simulink model "Refined_Model_230322"  (R2020b)
settings: Solver=FixedStepAuto  StartTime=0.0  StopTime=90  FixedStep=dt  RelTol=1e-3
values from neighbouring files (symbols this model uses):
  CovDist = RoadProfile(:,4)    [ICE_Val.m]
  Cx = VehicleDefine(7,3)    [BEV_Basictest.m]    (also in GPS_val.m; ICEBEV_Script.m; ICEBEV_Script_VECTO.m; ICE_Script.m)
  Dist = 1:length(MaxSpeedProfile)    [GPS_val.m]    (also in ICE_Script.m; ICE_Val.m = [1:CovDist(end)])
  dt = 0.1    [GPS_val.m]    (also in ICEBEV_Script.m; ICEBEV_Script_VECTO.m; ICE_Script.m; ICE_Script_SSVal.m)
  DynRolRad = VehicleDefine(5,3)    [BEV_Basictest.m]    (also in GPS_val.m; ICEBEV_Script.m; ICEBEV_Script_VECTO.m; ICE_Script.m)
  EngineRpm = round(IntpTorCur(:,1))    [GPS_val.m]    (also in ICEBEV_Script.m; ICEBEV_Script_VECTO.m; ICE_Script.m; ICE_Script_SSVal.m)
  EngineRpmUse = [EngineRpmUse1; EngineRpmUse2]    [GPS_val.m]    (also in ICEBEV_Script.m; ICEBEV_Script_VECTO.m; ICE_Script.m; ICE_Script_SSVal.m)
  etaClutch = VehicleDefine(23,3)    [GPS_val.m]    (also in ICEBEV_Script.m; ICEBEV_Script_VECTO.m; ICE_Script.m; ICE_Script_SSVal.m)
  etaGRa = GBXDefine(:,3)    [GPS_val.m]    (also in ICEBEV_Script.m; ICEBEV_Script_VECTO.m; ICE_Script.m; ICE_Script_SSVal.m)
  FDR = VehicleDefine(20,3)    [BEV_Basictest.m]    (also in GPS_val.m = VehicleDefine(22,3); ICEBEV_Script.m = VehicleDefine(22,3); ICEBEV_Script_VECTO.m = VehicleDefine(22,3); ICE_Script.m = VehicleDefine(22,3))
  FLoadTor = IntpTorCur(:,2)    [GPS_val.m]    (also in ICEBEV_Script.m; ICEBEV_Script_VECTO.m; ICE_Script.m; ICE_Script_SSVal.m)
  Fr = VehicleDefine(13,3)    [BEV_Basictest.m]    (also in GPS_val.m; ICEBEV_Script.m; ICEBEV_Script_VECTO.m; ICE_Script.m)
  g = VehicleDefine(14,3)    [BEV_Basictest.m]    (also in GPS_val.m; ICEBEV_Script.m; ICEBEV_Script_VECTO.m; ICE_Script.m)
  GNo = GBXDefine(:,1)    [GPS_val.m]    (also in ICEBEV_Script.m; ICEBEV_Script_VECTO.m; ICE_Script.m; ICE_Script_SSVal.m)
  GRa = GBXDefine(:,2)    [GPS_val.m]    (also in ICEBEV_Script.m; ICEBEV_Script_VECTO.m; ICE_Script.m; ICE_Script_SSVal.m)
  IntpSlope = round(IntpSlope,1)    [GPS_val.m]    (also in ICE_Script.m; ICE_Val.m = A)
  Jk = VehicleDefine(15,3)    [BEV_Basictest.m]    (also in GPS_val.m; ICEBEV_Script.m; ICEBEV_Script_VECTO.m; ICE_Script.m)
  Jm = VehicleDefine(16,3)    [GPS_val.m]    (also in ICEBEV_Script.m; ICEBEV_Script_VECTO.m; ICE_Script.m; ICE_Script_SSVal.m)
  MaxSpeedProfile = FMSP    [GPS_val.m]    (also in ICE_Script.m; ICE_Val.m = repelem(SegSPLatinmps,SegLeninm))
  Me = VehicleDefine(10,3)    [BEV_Basictest.m]    (also in GPS_val.m; ICEBEV_Script.m; ICEBEV_Script_VECTO.m; ICE_Script.m)
  MotoringTor = IntpTorCur(:,3)    [GPS_val.m]    (also in ICEBEV_Script.m; ICEBEV_Script_VECTO.m; ICE_Script.m; ICE_Script_SSVal.m)
  Mt = VehicleDefine(12,3)    [BEV_Basictest.m]    (also in GPS_val.m; ICEBEV_Script.m; ICEBEV_Script_VECTO.m; ICE_Script.m)
  Mtot = Mv+Me+Mt    [BEV_Basictest.m]    (also in GPS_val.m; ICEBEV_Script.m; ICEBEV_Script_VECTO.m; ICE_Script.m)
  Mv = VehicleDefine(9,3)    [BEV_Basictest.m]    (also in GPS_val.m; ICEBEV_Script.m; ICEBEV_Script_VECTO.m; ICE_Script.m)
  NoWhlFA = VehicleDefine(2,3)    [BEV_Basictest.m]    (also in GPS_val.m; ICE_Script.m; ICE_Val.m; ICE_Val_new.m)
  NoWhlRA = VehicleDefine(4,3)    [BEV_Basictest.m]    (also in GPS_val.m; ICE_Script.m; ICE_Val.m; ICE_Val_new.m)
  rho = VehicleDefine(6,3)    [BEV_Basictest.m]    (also in GPS_val.m; ICEBEV_Script.m; ICEBEV_Script_VECTO.m; ICE_Script.m)
  SegNo = RoadProfile(:,1)    [ICE_Val.m]
  SegSPLatinmps = (sqrt(aMaxLat*g*CurRadinm))    [GPS_val.m]    (also in ICE_Script.m; ICE_Val.m)
  Sx = VehicleDefine(8,3)    [BEV_Basictest.m]    (also in GPS_val.m; ICEBEV_Script.m; ICEBEV_Script_VECTO.m; ICE_Script.m)
undefined symbols (not defined in the file or in its folder): AccLim, FLoadTorUse, G1Inprpm, GearNo, GInprpm, GInpTor, GTorLoss, MaxSpinG, MaxWhlTorinG
libraries: pid_lib x1
settings Model: Creator=Kshitij  LastModifiedBy=Kshitij
settings SolverCC: AlgebraicLoopSolver=LineSearch

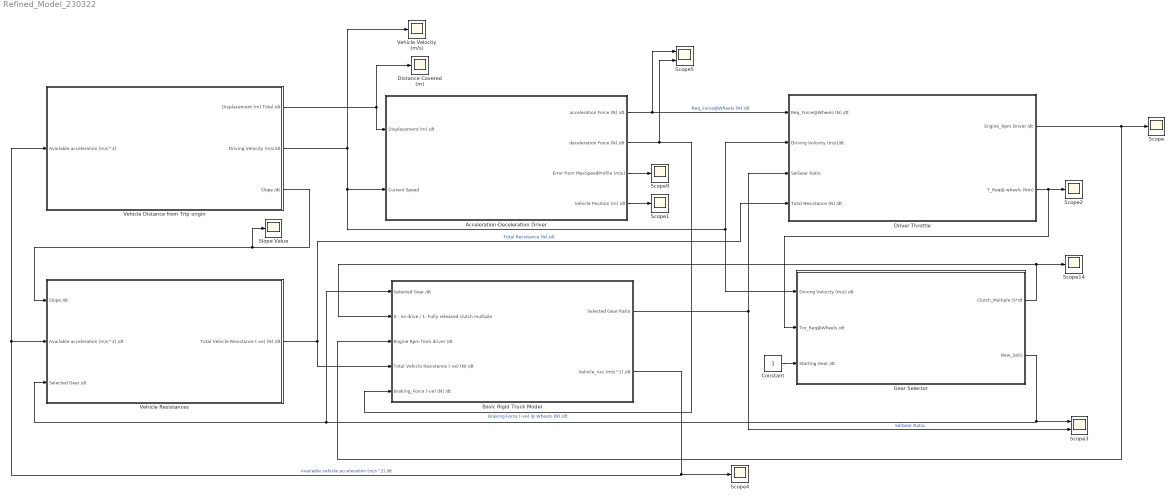
== system Refined_Model_230322 ==
  Acceleration-Deceleration Driver : Subsystem
  Basic Rigid Truck Model : Subsystem
  Constant : Constant
  Distance Covered (m) : Scope
  Driver Throttle : Subsystem
  Gear Selector : Subsystem
  Scope{,1..2,4,9,14} (6 alike) : Scope
  Scope3 : Scope  NumInputPorts=2
  Scope5 : Scope  NumInputPorts=2
  Slope Value : Scope
  Vehicle Distance from Trip origin : Subsystem
  Vehicle Resistances : Subsystem
  Vehicle Velocity (m/s) : Scope
  wires:
  Vehicle Distance from Trip origin/1(Displacement (m) Total /dt) -> Distance Covered (m)/1, Acceleration-Deceleration Driver/1(Displacement (m) /dt)
  Vehicle Resistances/1(Total Vehicle Resistance (-ve) (N) /dt) -> Basic Rigid Truck Model/4(Total Vehicle Resistance (-ve) (N) /dt), Driver Throttle/4(Total Resistance (N) /dt)  "Total Resistance (N) /dt"
  Basic Rigid Truck Model/2(Vehicle_Acc (m/s^2) /dt) -> Vehicle Distance from Trip origin/1(Available acceleration (m/s^2)), Vehicle Resistances/2(Available acceleration (m/s^2) /dt), Scope4/1  "Available vehicle acceleration (m/s^2) /dt"
  Vehicle Distance from Trip origin/3(Slope /dt) -> Vehicle Resistances/1(Slope /dt), Slope Value/1
  Gear Selector/1(Clutch_Multiple /5*dt) -> Scope14/1, Basic Rigid Truck Model/2(0 - no drive / 1- Fully released clutch multiple)
  Gear Selector/2(New_SelG) -> Vehicle Resistances/3(Selected Gear /dt), Basic Rigid Truck Model/1(Selected Gear /dt), Scope3/1
  Acceleration-Deceleration Driver/3(Error from MaxSpeedProfile (m/s)) -> Scope9/1
  Acceleration-Deceleration Driver/2(deceleration Force (N) /dt) -> Scope5/2, Basic Rigid Truck Model/5(Braking_Force (-ve) (N) /dt)  "Braking Force (-ve) @ Wheels (N) /dt"
  Basic Rigid Truck Model/1(Selected Gear Ratio) -> Scope3/2, Driver Throttle/3(SelGear Ratio)  "SelGear Ratio"
  Acceleration-Deceleration Driver/1(acceleration Force (N) /dt) -> Scope5/1, Driver Throttle/1(Req_Force@Wheels (N) /dt)  "Req_Force@Wheels (N) /dt"
  Constant/1 -> Gear Selector/3(Starting Gear /dt)
  Driver Throttle/1(Engine_Rpm Driver /dt) -> Scope/1, Basic Rigid Truck Model/3(Engine Rpm from driver /dt)
  Driver Throttle/2(T_Req@ wheels (Nm)) -> Gear Selector/2(Tor_Req@Wheels /dt), Scope2/1
  Acceleration-Deceleration Driver/4(Vehicle Position (m) /dt) -> Scope1/1
  Vehicle Distance from Trip origin/2(Driving Velocity (m/s)dt) -> Vehicle Velocity (m/s)/1, Acceleration-Deceleration Driver/2(Current Speed), Gear Selector/1(Driving Velocity (m/s) /dt), Driver Throttle/2(Driving Velocity (m/s)/dt)

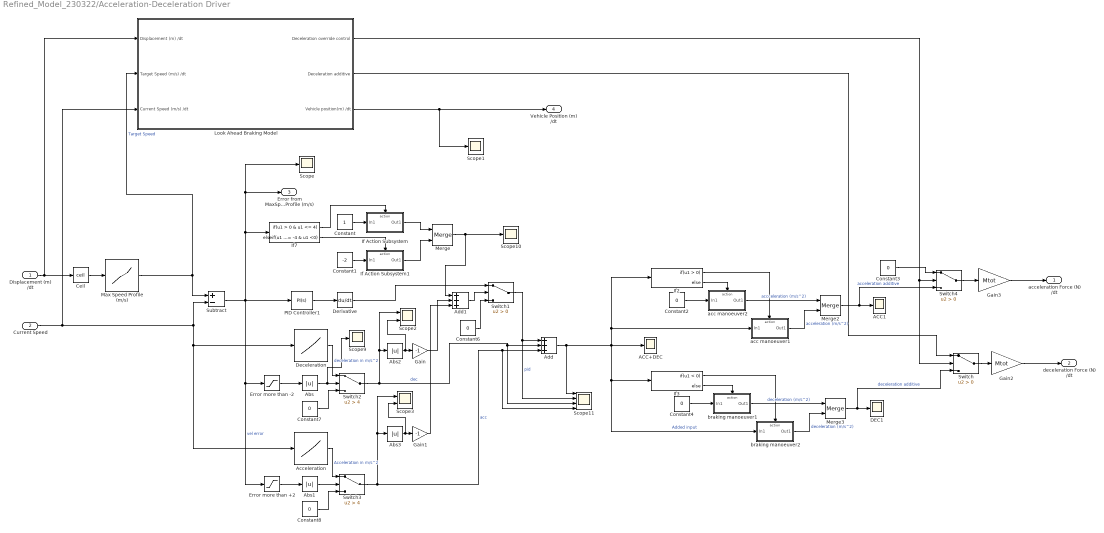
== system Refined_Model_230322/Acceleration-Deceleration Driver ==
  Displacement (m) /dt : Inport
  Current Speed : Inport  Port=2
  ACC+DEC : Scope
  ACC1 : Scope
  Abs{,1..3} (4 alike) : Abs
  Acceleration : Lookup_n-D  NumberOfTableDimensions=1  BreakpointsForDimension1=AccLim(:,1)  Table=AccLim(:,2)  InternalRulePriority=Speed  RndMeth=Simplest  InputSameDT=on
  Add : Sum  Inputs=+++
  Add1 : Sum  Inputs=+++
  Ceil : Rounding  Operator=ceil
  Constant : Constant
  Constant1 : Constant  Value=-2
  Constant{2..4,6..8} (6 alike) : Constant  Value=0
  DEC1 : Scope
  Deceleration : Lookup_n-D  NumberOfTableDimensions=1  BreakpointsForDimension1=AccLim(:,1)  Table=AccLim(:,3)  InternalRulePriority=Speed  RndMeth=Simplest  InputSameDT=on
  Derivative : Derivative
  Error more than +2 : Saturate  UpperLimit=inf  LowerLimit=4
  Error more than -2 : Saturate  UpperLimit=-4  LowerLimit=-inf
  Gain : Gain  Gain=-1
  Gain1 : Gain  Gain=-1
  Gain2 : Gain  Gain=Mtot
  Gain3 : Gain  Gain=Mtot
  If Action Subsystem : Subsystem  TreatAsAtomicUnit=on
  If Action Subsystem1 : Subsystem  TreatAsAtomicUnit=on
  If2 : If
  If3 : If  IfExpression=u1 < 0
  If7 : If  IfExpression=u1 > 0 & u1 <= 4  ElseIfExpressions=u1 >= -4 & u1 <0  ShowElse=off
  Look Ahead Braking Model : Subsystem
  Max Speed Profile (m/s) : Lookup_n-D  NumberOfTableDimensions=1  BreakpointsForDimension1=[1:length(MaxSpeedProfile)]  BreakpointsForDimension2=G1Inprpm  Table=MaxSpeedProfile  InterpMethod=Linear Lagrange  InternalRulePriority=Speed  RndMeth=Simplest  InputSameDT=on
  Merge : Merge
  Merge2 : Merge
  Merge3 : Merge
  PID Controller1 : pid_lib/PID Controller  Controller=PI  Form=Parallel  TimeDomain=Continuous-time  UseExternalTs=off  SampleTime=-1  IntegratorMethod=Forward Euler  FilterMethod=Forward Euler  ControllerParametersSource=internal  P=0.024  I=0.28  D=0.2  UseFilter=on  N=100  TunerSelectOption=Frequency Response Based  InitialConditionSource=internal  InitialConditionForIntegrator=0  InitialConditionForFilter=0  DifferentiatorICPrevScaledInput=0  ExternalReset=none  TrackingMode=off  Kt=1  LimitOutput=off  SatLimitsSource=internal  UpperSaturationLimit=inf  LowerSaturationLimit=-inf  LinearizeAsGain=on  AntiWindupMode=none  Kb=1  POutMin=[]  POutMax=[]  IOutMin=[]  IOutMax=[]  DOutMin=[]  DOutMax=[]  NOutMin=[]  NOutMax=[]  SumOutMin=[]  SumOutMax=[]  SaturationOutMin=[]  SaturationOutMax=[]  PParamMin=[]  PParamMax=[]  IParamMin=[]  IParamMax=[]  DParamMin=[]  DParamMax=[]  NParamMin=[]  NParamMax=[]  KbParamMin=[]  KbParamMax=[]  KtParamMin=[]  KtParamMax=[]  KbOutMin=[]  KbOutMax=[]  KtOutMin=[]  KtOutMax=[]  IntegratorOutMin=[]  IntegratorOutMax=[]  FilterOutMin=[]  FilterOutMax=[]  SumI1OutMin=[]  SumI1OutMax=[]  SumI2OutMin=[]  SumI2OutMax=[]  SumI3OutMin=[]  SumI3OutMax=[]  SumI4OutMin=[]  SumI4OutMax=[]  SumDOutMin=[]  SumDOutMax=[]  DifferentiatorOutMin=[]  DifferentiatorOutMax=[]  FilterDiffOutCoefMin=[]  FilterDiffOutCoefMax=[]  ReciprocalOutMin=[]  ReciprocalOutMax=[]  SumDenOutMin=[]  SumDenOutMax=[]  SumNumOutMin=[]  SumNumOutMax=[]  DivideOutMin=[]  DivideOutMax=[]  UdiffTsProdOutMin=[]  UdiffTsProdOutMax=[]  NTsProdOutMin=[]  NTsProdOutMax=[]  UintegralTsProdOutMin=[]  UintegralTsProdOutMax=[]  UngainTsProdOutMin=[]  UngainTsProdOutMax=[]  IntegratorContinuousStateAttributes=''  IntegratorStateMustResolveToSignalObject=off  IntegratorRTWStateStorageClass=Auto  FilterContinuousStateAttributes=''  FilterStateMustResolveToSignalObject=off  FilterRTWStateStorageClass=Auto  ParallelPVariant=InternalParameters  IdealPVariant=Disabled  IVariant=InternalParameters  DVariant=Disabled  IntegratorVariant=Continuous  SatVariant=Disabled  AWVariant=Passthrough  PCopyVariant=Disabled  TRVariant=Disabled  FdbkBlocksVariant=Forward  IdealPFdbkVariant=Disabled  SatFdbkVariant=Disabled  DerivativeFilterVariant=Disabled  NVariant=Disabled  NCopyVariant=Disabled_SignalSpec  FilterICVariant=Disabled  IntegratorICVariant=InternalICs  ExternalResetVariant=Disabled  TRSumVariant=Passthrough  SumFdbkVariant=Disabled  SumVariant=Sum_PI  TsampFilterVariant=InternalTs  TsampNgainVariant=Passthrough  TsampIntegralVariant=Passthrough  ExternalSaturationOutDataTypeStr=Inherit: Same as second input
  Scope{,1,9..10} (4 alike) : Scope
  Scope11 : Scope  NumInputPorts=4
  Scope2 : Scope  NumInputPorts=2
  Scope3 : Scope  NumInputPorts=2
  Subtract : Sum  Inputs=+-
  Switch : Switch  Criteria=u2 > Threshold
  Switch1 : Switch  Criteria=u2 > Threshold
  Switch2 : Switch  Criteria=u2 > Threshold  Threshold=4
  Switch3 : Switch  Criteria=u2 > Threshold  Threshold=4
  Switch4 : Switch  Criteria=u2 > Threshold
  acc manoeuver1 : Subsystem  TreatAsAtomicUnit=on
  acc manoeuver2 : Subsystem  TreatAsAtomicUnit=on
  braking manoeuver1 : Subsystem  TreatAsAtomicUnit=on
  braking manoeuver2 : Subsystem  TreatAsAtomicUnit=on
  acceleration Force (N) /dt : Outport
  deceleration Force (N) /dt : Outport  Port=2
  Error from MaxSpeedProfile (m/s) : Outport  Port=3
  Vehicle Position (m) /dt : Outport  Port=4
  wires:
  Merge2/1 -> Switch4/3, ACC1/1  "acceleration additive"
  Merge3/1 -> Switch/3, DEC1/1  "deceleration additive"
  Max Speed Profile (m/s)/1 -> Look Ahead Braking Model/2(Target Speed (m/s) /dt), Subtract/1  "Target Speed"
  Displacement (m) /dt/1 -> Look Ahead Braking Model/1(Displacement (m) /dt), Ceil/1
  Look Ahead Braking Model/1(Deceleration override control) -> Switch/2, Switch4/2
  Look Ahead Braking Model/2(Deceleration additive) -> Switch/1
  Switch/1 -> Gain2/1
  If2/1 -> acc manoeuver1/Action
  acc manoeuver2/1(Out1) -> Merge2/1  "accceleration (m/s^2)"
  Constant2/1 -> acc manoeuver2/1(In1)
  If2/2 -> acc manoeuver2/Action
  acc manoeuver1/1(Out1) -> Merge2/2  "acceleration (m/s^2)"
  Constant4/1 -> braking manoeuver1/1(In1)
  braking manoeuver2/1(Out1) -> Merge3/2  "deceleration (m/s^2)"
  If3/1 -> braking manoeuver2/Action
  If3/2 -> braking manoeuver1/Action
  braking manoeuver1/1(Out1) -> Merge3/1  "deceleration (m/s^2)"
  Switch3/1 -> Scope3/1, Abs3/1, Scope11/4, Add/3  "acc"
  Acceleration/1 -> Switch3/1  "Acceleration in m/s^2"
  Error more than -2/1 -> Abs/1
  Current Speed/1 -> Subtract/2, Acceleration/1, Deceleration/1, Look Ahead Braking Model/3(Current Speed (m/s) /dt)
  PID Controller1/1 -> Derivative/1
  Constant8/1 -> Switch3/3
  Deceleration/1 -> Switch2/1  "deceleration in m/s^2"
  Add1/1 -> Switch1/2
  Abs/1 -> Scope9/1, Switch2/2
  Gain/1 -> Add1/2
  Constant6/1 -> Switch1/3
  Abs3/1 -> Scope3/2, Gain1/1
  If7/1 -> If Action Subsystem/Action
  Switch1/1 -> Add/1, Scope11/2  "pid"
  Constant7/1 -> Switch2/3
  Constant/1 -> If Action Subsystem/1(In1)
  Abs2/1 -> Scope2/2, Gain/1
  Switch2/1 -> Scope2/1, Abs2/1, Scope11/3, Add/2  "dec"
  Abs1/1 -> Switch3/2
  Subtract/1 -> PID Controller1/1, Scope/1, Error from MaxSpeedProfile (m/s)/1, If7/1, Error more than +2/1, Error more than -2/1  "vel error"
  Gain1/1 -> Add1/3
  Add/1 -> If3/1, braking manoeuver2/1(In1), ACC+DEC/1, If2/1, acc manoeuver1/1(In1), Scope11/1  "Added input"
  Error more than +2/1 -> Abs1/1
  Ceil/1 -> Max Speed Profile (m/s)/1
  If7/2 -> If Action Subsystem1/Action
  Constant1/1 -> If Action Subsystem1/1(In1)
  If Action Subsystem1/1(Out1) -> Merge/2
  If Action Subsystem/1(Out1) -> Merge/1
  Merge/1 -> Add1/1, Scope10/1
  Constant3/1 -> Switch4/1
  Switch4/1 -> Gain3/1
  Gain3/1 -> acceleration Force (N) /dt/1
  Gain2/1 -> deceleration Force (N) /dt/1
  Derivative/1 -> Switch1/1
  Look Ahead Braking Model/3(Vehicle position(m) /dt) -> Scope1/1, Vehicle Position (m) /dt/1

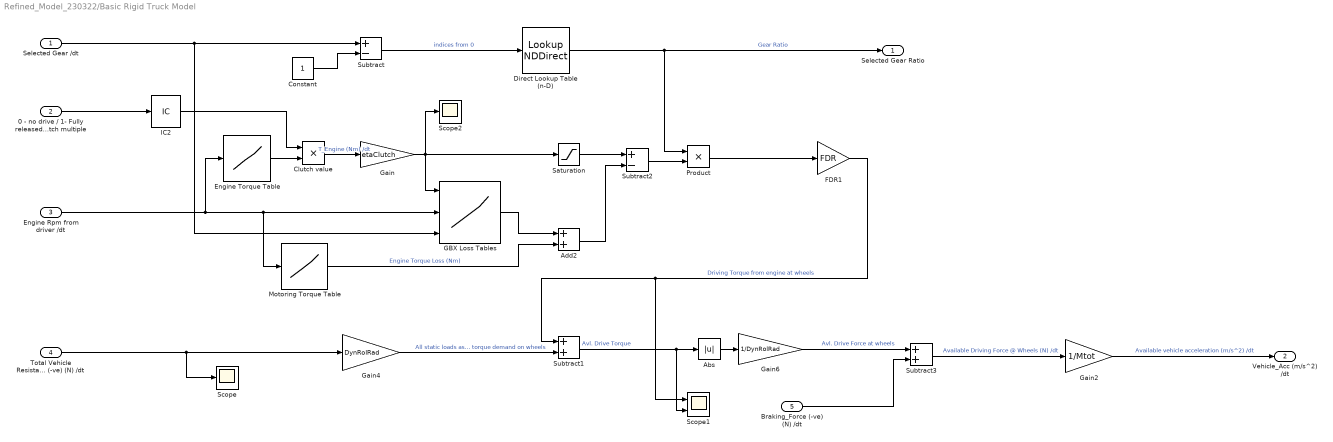
== system Refined_Model_230322/Basic Rigid Truck Model ==
  Selected Gear /dt : Inport
  0 - no drive / 1- Fully released clutch multiple : Inport  Port=2
  Engine Rpm from driver /dt : Inport  Port=3
  Total Vehicle Resistance (-ve) (N) /dt : Inport  Port=4
  Braking_Force (-ve) (N) /dt : Inport  Port=5
  Abs : Abs
  Add2 : Sum
  Clutch value : Product
  Constant : Constant
  Direct Lookup Table (n-D) : LookupNDDirect  NumberOfTableDimensions=1  Table=GRa
  Engine Torque Table : Lookup_n-D  NumberOfTableDimensions=1  BreakpointsForDimension1=EngineRpm  BreakpointsForDimension2=G1Inprpm  Table=FLoadTor  InterpMethod=Linear Lagrange  InternalRulePriority=Speed  RndMeth=Simplest  InputSameDT=on
  FDR1 : Gain  Gain=FDR
  GBX Loss Tables : Lookup_n-D  NumberOfTableDimensions=3  BreakpointsForDimension1=GInpTor  BreakpointsForDimension2=GInprpm  BreakpointsForDimension3=GearNo  Table=GTorLoss  InterpMethod=Linear Lagrange  InternalRulePriority=Speed  RndMeth=Simplest  InputSameDT=on
      settings: InputPortMap=u0,u1,u2
  Gain : Gain  Gain=etaClutch
  Gain2 : Gain  Gain=1/Mtot
  Gain4 : Gain  Gain=DynRolRad
  Gain6 : Gain  Gain=1/DynRolRad
  IC2 : InitialCondition
  Motoring Torque Table : Lookup_n-D  NumberOfTableDimensions=1  BreakpointsForDimension1=EngineRpm  BreakpointsForDimension2=G1Inprpm  Table=MotoringTor  InterpMethod=Linear Lagrange  InternalRulePriority=Speed  RndMeth=Simplest  InputSameDT=on
  Product : Product
  Saturation : Saturate  UpperLimit=max(FLoadTorUse)  LowerLimit=min(FLoadTorUse)
  Scope : Scope
  Scope1 : Scope  NumInputPorts=2
  Scope2 : Scope
  Subtract : Sum  Inputs=+-
  Subtract1 : Sum
  Subtract2 : Sum  Inputs=+-
  Subtract3 : Sum
  Selected Gear Ratio : Outport
  Vehicle_Acc (m/s^2) /dt : Outport  Port=2
  wires:
  GBX Loss Tables/1 -> Add2/1
  Motoring Torque Table/1 -> Add2/2  "Engine Torque Loss (Nm)"
  FDR1/1 -> Scope1/1, Subtract1/1  "Driving Torque from engine at wheels"
  Direct Lookup Table (n-D)/1 -> Selected Gear Ratio/1, Product/1  "Gear Ratio"
  Clutch value/1 -> Gain/1  "T_Engine (Nm) /dt"
  Gain4/1 -> Subtract1/2  "All static loads as torque demand on wheels"
  Subtract1/1 -> Abs/1, Scope1/2  "Avl. Drive Torque"
  Add2/1 -> Subtract2/2
  Subtract2/1 -> Product/2
  0 - no drive / 1- Fully released clutch multiple/1 -> IC2/1
  Total Vehicle Resistance (-ve) (N) /dt/1 -> Scope/1, Gain4/1
  Gain6/1 -> Subtract3/1  "Avl. Drive Force at wheels"
  Saturation/1 -> Subtract2/1
  Selected Gear /dt/1 -> Subtract/1, GBX Loss Tables/3
  Subtract/1 -> Direct Lookup Table (n-D)/1  "indices from 0"
  Constant/1 -> Subtract/2
  IC2/1 -> Clutch value/1
  Subtract3/1 -> Gain2/1  "Available Driving Force @ Wheels (N) /dt"
  Gain2/1 -> Vehicle_Acc (m/s^2) /dt/1  "Available vehicle acceleration (m/s^2) /dt"
  Braking_Force (-ve) (N) /dt/1 -> Subtract3/2
  Abs/1 -> Gain6/1
  Engine Rpm from driver /dt/1 -> GBX Loss Tables/2, Motoring Torque Table/1, Engine Torque Table/1
  Engine Torque Table/1 -> Clutch value/2
  Product/1 -> FDR1/1
  Gain/1 -> Saturation/1, Scope2/1, GBX Loss Tables/1

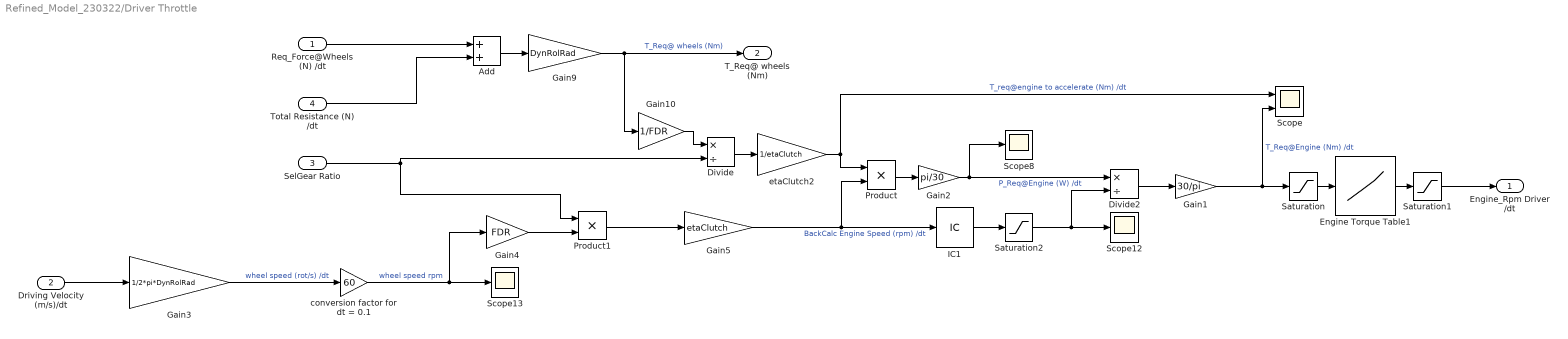
== system Refined_Model_230322/Driver Throttle ==
  Req_Force@Wheels (N) /dt : Inport
  Driving Velocity (m/s)/dt : Inport  Port=2
  SelGear Ratio : Inport  Port=3
  Total Resistance (N) /dt : Inport  Port=4
  Add : Sum
  Divide : Product  Inputs=*/
  Divide2 : Product  Inputs=*/
  Engine Torque Table1 : Lookup_n-D  NumberOfTableDimensions=1  BreakpointsForDimension1=FLoadTorUse  BreakpointsForDimension2=G1Inprpm  Table=EngineRpmUse  InterpMethod=Linear Lagrange  InternalRulePriority=Speed  RndMeth=Simplest  InputSameDT=on
  Gain1 : Gain  Gain=30/pi
  Gain10 : Gain  Gain=1/FDR
  Gain2 : Gain  Gain=pi/30
  Gain3 : Gain  Gain=1/2*pi*DynRolRad
  Gain4 : Gain  Gain=FDR
  Gain5 : Gain  Gain=etaClutch
  Gain9 : Gain  Gain=DynRolRad
  IC1 : InitialCondition  Value=0.1
  Product : Product
  Product1 : Product
  Saturation : Saturate  UpperLimit=max(FLoadTorUse)  LowerLimit=min(FLoadTorUse)
  Saturation1 : Saturate  UpperLimit=max(EngineRpmUse)  LowerLimit=min(EngineRpmUse)
  Saturation2 : Saturate  UpperLimit=max(EngineRpmUse)  LowerLimit=0
  Scope : Scope  NumInputPorts=2
  Scope12 : Scope
  Scope13 : Scope
  Scope8 : Scope
  conversion factor for dt = 0.1 : Gain  Gain=60
  etaClutch2 : Gain  Gain=1/etaClutch
  Engine_Rpm Driver /dt : Outport
  T_Req@ wheels (Nm) : Outport  Port=2
  wires:
  etaClutch2/1 -> Scope/1, Product/1  "T_req@engine to accelerate (Nm) /dt"
  Product/1 -> Gain2/1
  conversion factor for dt = 0.1/1 -> Scope13/1, Gain4/1  "wheel speed rpm"
  Engine Torque Table1/1 -> Saturation1/1
  Add/1 -> Gain9/1
  Gain4/1 -> Product1/2
  Gain2/1 -> Scope8/1, Divide2/1  "P_Req@Engine (W) /dt"
  Saturation2/1 -> Scope12/1, Divide2/2
  Gain9/1 -> Gain10/1, T_Req@ wheels (Nm)/1  "T_Req@ wheels (Nm)"
  Gain5/1 -> IC1/1, Product/2  "BackCalc Engine Speed (rpm) /dt"
  Gain3/1 -> conversion factor for dt = 0.1/1  "wheel speed (rot/s) /dt"
  Gain10/1 -> Divide/1
  Divide2/1 -> Gain1/1
  Gain1/1 -> Scope/2, Saturation/1  "T_Req@Engine (Nm) /dt"
  SelGear Ratio/1 -> Divide/2, Product1/1
  IC1/1 -> Saturation2/1
  Product1/1 -> Gain5/1
  Saturation1/1 -> Engine_Rpm Driver /dt/1
  Req_Force@Wheels (N) /dt/1 -> Add/1
  Saturation/1 -> Engine Torque Table1/1
  Driving Velocity (m/s)/dt/1 -> Gain3/1
  Divide/1 -> etaClutch2/1
  Total Resistance (N) /dt/1 -> Add/2

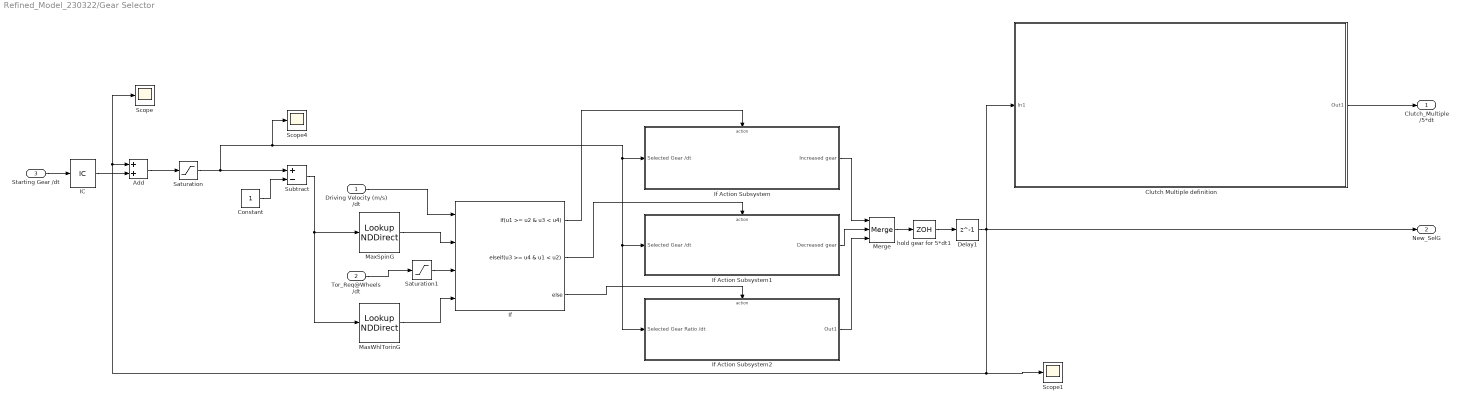
== system Refined_Model_230322/Gear Selector ==
  Driving Velocity (m/s) /dt : Inport
  Tor_Req@Wheels /dt : Inport  Port=2
  Starting Gear /dt : Inport  Port=3
  Add : Sum
  Clutch Multiple definition : Subsystem
  Constant : Constant
  Delay1 : Delay  DelayLength=1
  IC : InitialCondition
  If : If  NumInputs=4  IfExpression=u1 >= u2 & u3 < u4  ElseIfExpressions=u3 >= u4 & u1 < u2
  If Action Subsystem : Subsystem  TreatAsAtomicUnit=on
  If Action Subsystem1 : Subsystem  TreatAsAtomicUnit=on
  If Action Subsystem2 : Subsystem  TreatAsAtomicUnit=on
  MaxSpinG : LookupNDDirect  NumberOfTableDimensions=1  Table=MaxSpinG
  MaxWhlTorinG : LookupNDDirect  NumberOfTableDimensions=1  Table=MaxWhlTorinG
  Merge : Merge  Inputs=3
  Saturation : Saturate  UpperLimit=max(GNo)  LowerLimit=0
  Saturation1 : Saturate  UpperLimit=max(MaxWhlTorinG)  LowerLimit=0
  Scope : Scope
  Scope1 : Scope
  Scope4 : Scope
  Subtract : Sum  Inputs=+-
  hold gear for 5*dt1 : ZeroOrderHold  SampleTime=10*dt
  Clutch_Multiple /5*dt : Outport
  New_SelG : Outport  Port=2
  wires:
  If/1 -> If Action Subsystem/Action
  MaxWhlTorinG/1 -> If/4
  Driving Velocity (m/s) /dt/1 -> If/1
  MaxSpinG/1 -> If/2
  Tor_Req@Wheels /dt/1 -> Saturation1/1
  If/2 -> If Action Subsystem1/Action
  If Action Subsystem/1(Increased gear) -> Merge/1
  If Action Subsystem1/1(Decreased gear) -> Merge/2
  Constant/1 -> Subtract/2
  Subtract/1 -> MaxSpinG/1, MaxWhlTorinG/1
  If/3 -> If Action Subsystem2/Action
  If Action Subsystem2/1(Out1) -> Merge/3
  Add/1 -> Saturation/1
  Merge/1 -> hold gear for 5*dt1/1
  Saturation/1 -> Subtract/1, If Action Subsystem2/1(Selected Gear Ratio /dt), If Action Subsystem1/1(Selected Gear /dt), If Action Subsystem/1(Selected Gear /dt), Scope4/1
  Starting Gear /dt/1 -> IC/1
  IC/1 -> Add/2
  hold gear for 5*dt1/1 -> Delay1/1
  Saturation1/1 -> If/3
  Delay1/1 -> Clutch Multiple definition/1(In1), New_SelG/1, Scope/1, Add/1, Scope1/1
  Clutch Multiple definition/1(Out1) -> Clutch_Multiple /5*dt/1

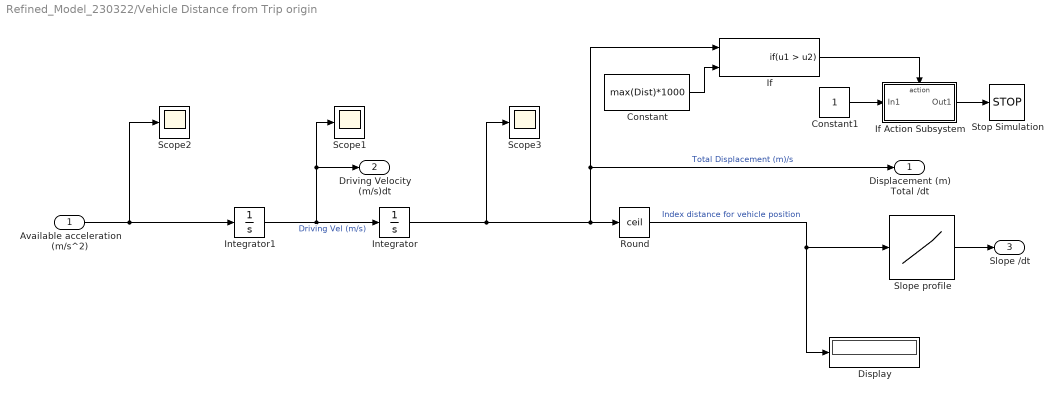
== system Refined_Model_230322/Vehicle Distance from Trip origin ==
  Available acceleration (m/s^2) : Inport
  Constant : Constant  Value=max(Dist)*1000
  Constant1 : Constant
  Display : Display
  If : If  NumInputs=2  IfExpression=u1 > u2  ShowElse=off
  If Action Subsystem : Subsystem  TreatAsAtomicUnit=on
  Integrator : Integrator
  Integrator1 : Integrator
  Round : Rounding  Operator=ceil
  Scope1 : Scope
  Scope2 : Scope
  Scope3 : Scope
  Slope profile : Lookup_n-D  NumberOfTableDimensions=1  BreakpointsForDimension1=1: length(IntpSlope)  Table=IntpSlope  InternalRulePriority=Speed  RndMeth=Simplest  InputSameDT=on
  Stop Simulation : Stop
  Displacement (m) Total /dt : Outport
  Driving Velocity (m/s)dt : Outport  Port=2
  Slope /dt : Outport  Port=3
  wires:
  Integrator1/1 -> Scope1/1, Driving Velocity (m/s)dt/1, Integrator/1  "Driving Vel (m/s)"
  Integrator/1 -> Displacement (m) Total /dt/1, If/1, Round/1, Scope3/1  "Total Displacement (m)/s"
  Round/1 -> Display/1, Slope profile/1  "Index distance for vehicle position"
  Slope profile/1 -> Slope /dt/1
  Constant/1 -> If/2
  If/1 -> If Action Subsystem/Action
  If Action Subsystem/1(Out1) -> Stop Simulation/1
  Constant1/1 -> If Action Subsystem/1(In1)
  Available acceleration (m/s^2)/1 -> Scope2/1, Integrator1/1

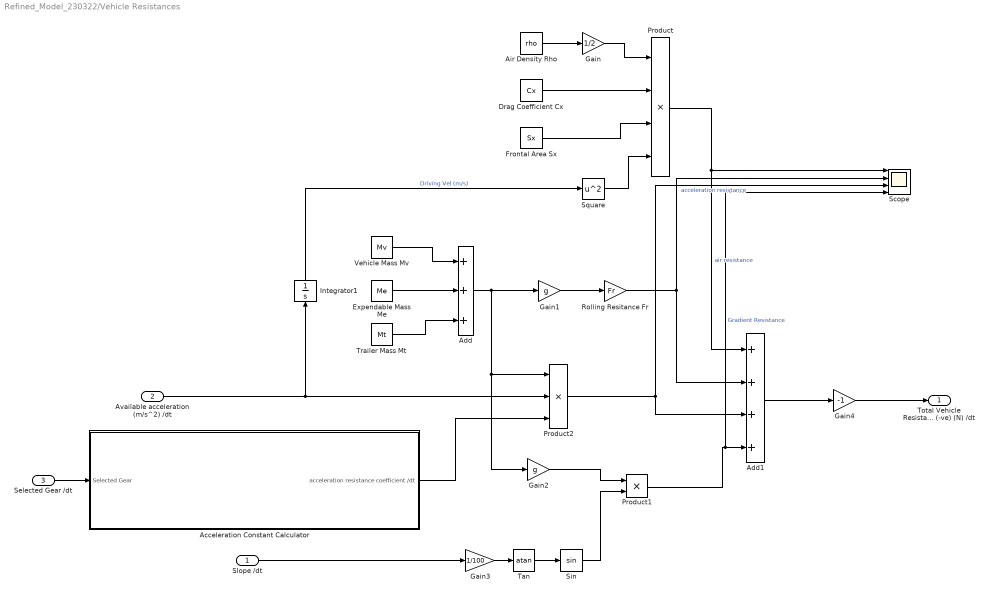
== system Refined_Model_230322/Vehicle Resistances ==
  Slope /dt : Inport
  Available acceleration (m/s^2) /dt : Inport  Port=2
  Selected Gear /dt : Inport  Port=3
  Acceleration Constant Calculator : Subsystem
  Add : Sum  Inputs=+++
  Add1 : Sum  Inputs=++++
  Air Density Rho : Constant  Value=rho
  Drag Coefficient Cx : Constant  Value=Cx
  Expendable Mass Me : Constant  Value=Me
  Frontal Area Sx : Constant  Value=Sx
  Gain : Gain  Gain=1/2
  Gain1 : Gain  Gain=g
  Gain2 : Gain  Gain=g
  Gain3 : Gain  Gain=1/100
  Gain4 : Gain  Gain=-1
  Integrator1 : Integrator
  Product : Product  Inputs=4
  Product1 : Product
  Product2 : Product  Inputs=3
  Rolling Resitance Fr : Gain  Gain=Fr
  Scope : Scope  NumInputPorts=4
  Sin : Trigonometry
  Square : Math  Operator=square  SaturateOnIntegerOverflow=on
  Tan : Trigonometry  Operator=atan
  Trailer Mass Mt : Constant  Value=Mt
  Vehicle Mass Mv : Constant  Value=Mv
  Total Vehicle Resistance (-ve) (N) /dt : Outport
  wires:
  Expendable Mass Me/1 -> Add/2
  Add/1 -> Gain2/1, Product2/1, Gain1/1
  Gain/1 -> Product/1
  Sin/1 -> Product1/2
  Tan/1 -> Sin/1
  Product1/1 -> Scope/4, Add1/4  "Gradient Resistance"
  Air Density Rho/1 -> Gain/1
  Drag Coefficient Cx/1 -> Product/2
  Integrator1/1 -> Square/1  "Driving Vel (m/s)"
  Slope /dt/1 -> Gain3/1
  Gain2/1 -> Product1/1
  Trailer Mass Mt/1 -> Add/3
  Rolling Resitance Fr/1 -> Scope/2, Add1/2
  Square/1 -> Product/4
  Gain1/1 -> Rolling Resitance Fr/1
  Vehicle Mass Mv/1 -> Add/1
  Product/1 -> Scope/1, Add1/1  "air resistance"
  Gain3/1 -> Tan/1
  Frontal Area Sx/1 -> Product/3
  Product2/1 -> Scope/3, Add1/3  "acceleration resistance"
  Acceleration Constant Calculator/1(acceleration resistance coefficient /dt) -> Product2/3
  Selected Gear /dt/1 -> Acceleration Constant Calculator/1(Selected Gear)
  Gain4/1 -> Total Vehicle Resistance (-ve) (N) /dt/1
  Add1/1 -> Gain4/1
  Available acceleration (m/s^2) /dt/1 -> Product2/2, Integrator1/1

== system Refined_Model_230322/Acceleration-Deceleration Driver/If Action Subsystem ==
  In1 : Inport
  Action Port : ActionPort  ActionPortLabel=if(u1 > 0 & u1 <= 4)
  Out1 : Outport
  wires:
  In1/1 -> Out1/1

== system Refined_Model_230322/Acceleration-Deceleration Driver/If Action Subsystem1 ==
  In1 : Inport
  Action Port : ActionPort  ActionPortLabel=elseif(u1 >= -4 & u1 <0)
  Out1 : Outport
  wires:
  In1/1 -> Out1/1

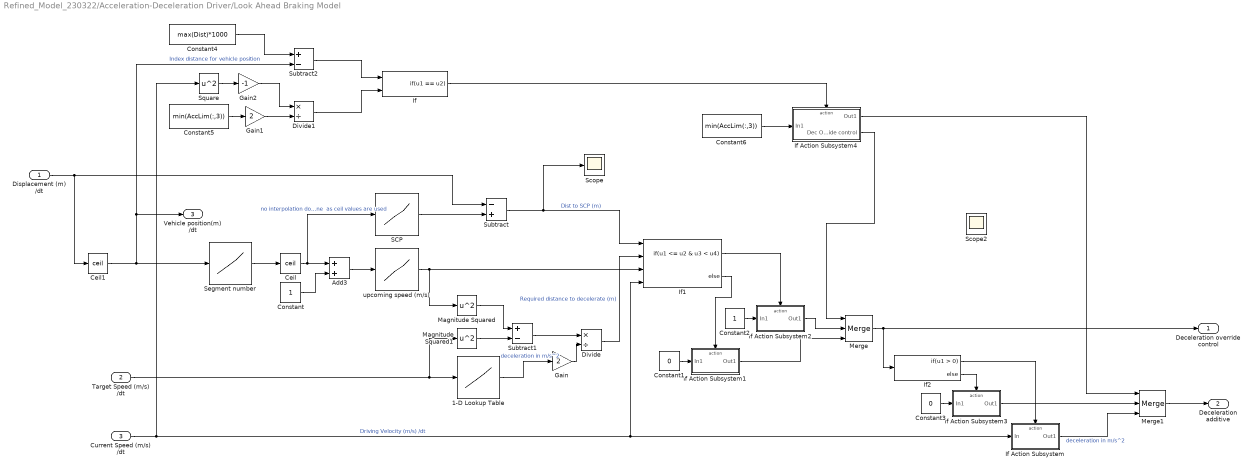
== system Refined_Model_230322/Acceleration-Deceleration Driver/Look Ahead Braking Model ==
  Displacement (m) /dt : Inport
  Target Speed (m/s) /dt : Inport  Port=2
  Current Speed (m/s) /dt : Inport  Port=3
  1-D Lookup Table : Lookup_n-D  NumberOfTableDimensions=1  BreakpointsForDimension1=AccLim(:,1)  Table=AccLim(:,3)  InternalRulePriority=Speed  RndMeth=Simplest  InputSameDT=on
  Add3 : Sum
  Ceil : Rounding  Operator=ceil
  Ceil1 : Rounding  Operator=ceil
  Constant : Constant
  Constant1 : Constant  Value=0
  Constant2 : Constant
  Constant3 : Constant  Value=0
  Constant4 : Constant  Value=max(Dist)*1000
  Constant5 : Constant  Value=min(AccLim(:,3))
  Constant6 : Constant  Value=min(AccLim(:,3))
  Divide : Product  Inputs=*/
  Divide1 : Product  Inputs=*/
  Gain : Gain  Gain=2
  Gain1 : Gain  Gain=2
  Gain2 : Gain  Gain=-1
  If : If  NumInputs=2  IfExpression=u1 == u2  ShowElse=off
  If Action Subsystem : Subsystem  TreatAsAtomicUnit=on
  If Action Subsystem1 : Subsystem  TreatAsAtomicUnit=on
  If Action Subsystem2 : Subsystem  TreatAsAtomicUnit=on
  If Action Subsystem3 : Subsystem  TreatAsAtomicUnit=on
  If Action Subsystem4 : Subsystem  TreatAsAtomicUnit=on
  If1 : If  NumInputs=4  IfExpression=u1 <= u2 & u3 < u4
  If2 : If
  Magnitude Squared : Math  Operator=square  SaturateOnIntegerOverflow=on
  Magnitude Squared1 : Math  Operator=square  SaturateOnIntegerOverflow=on
  Merge : Merge  Inputs=3
  Merge1 : Merge  Inputs=3
  SCP : Lookup_n-D  NumberOfTableDimensions=1  BreakpointsForDimension1=SegNo  BreakpointsForDimension2=G1Inprpm  Table=CovDist  InterpMethod=Linear Lagrange  InternalRulePriority=Speed  RndMeth=Simplest  InputSameDT=on
  Scope : Scope
  Scope2 : Scope
  Segment number : Lookup_n-D  NumberOfTableDimensions=1  BreakpointsForDimension1=CovDist  BreakpointsForDimension2=G1Inprpm  Table=SegNo  InterpMethod=Linear Lagrange  InternalRulePriority=Speed  RndMeth=Simplest  InputSameDT=on
  Square : Math  Operator=square  SaturateOnIntegerOverflow=on
  Subtract : Sum  Inputs=-+
  Subtract1 : Sum  Inputs=+-
  Subtract2 : Sum  Inputs=+-
  upcoming speed (m/s) : Lookup_n-D  NumberOfTableDimensions=1  BreakpointsForDimension1=SegNo  BreakpointsForDimension2=G1Inprpm  Table=SegSPLatinmps  InterpMethod=Linear Lagrange  InternalRulePriority=Speed  RndMeth=Simplest  InputSameDT=on
  Deceleration override control : Outport
  Deceleration additive : Outport  Port=2
  Vehicle position(m) /dt : Outport  Port=3
  wires:
  Displacement (m) /dt/1 -> Subtract/1, Ceil1/1
  Add3/1 -> upcoming speed (m/s)/1
  Ceil/1 -> SCP/1, Add3/1  "no interpolation done  as ceil values are used"
  SCP/1 -> Subtract/2
  upcoming speed (m/s)/1 -> If1/3, Magnitude Squared/1
  Constant/1 -> Add3/2
  Subtract/1 -> Scope/1, If1/1  "Dist to SCP (m)"
  Segment number/1 -> Ceil/1
  Ceil1/1 -> Subtract2/2, Vehicle position(m) /dt/1, Segment number/1  "Index distance for vehicle position"
  Magnitude Squared/1 -> Subtract1/1
  Target Speed (m/s) /dt/1 -> 1-D Lookup Table/1, Magnitude Squared1/1
  Subtract1/1 -> Divide/1
  Gain/1 -> Divide/2
  1-D Lookup Table/1 -> Gain/1  "deceleration in m/s^2"
  Divide/1 -> If1/2  "Required distance to decelerate (m)"
  Current Speed (m/s) /dt/1 -> Square/1, If Action Subsystem/1(In), If1/4  "Driving Velocity (m/s) /dt"
  If Action Subsystem/1(Out1) -> Merge1/3  "deceleration in m/s^2"
  If1/2 -> If Action Subsystem1/Action
  Constant1/1 -> If Action Subsystem1/1(In1)
  Constant2/1 -> If Action Subsystem2/1(In1)
  If1/1 -> If Action Subsystem2/Action
  If Action Subsystem2/1(Out1) -> Merge/2
  If Action Subsystem1/1(Out1) -> Merge/3
  Merge/1 -> Deceleration override control/1, If2/1
  If2/1 -> If Action Subsystem/Action
  If2/2 -> If Action Subsystem3/Action
  Constant3/1 -> If Action Subsystem3/1(In1)
  If Action Subsystem3/1(Out1) -> Merge1/2
  Merge1/1 -> Deceleration additive/1
  Magnitude Squared1/1 -> Subtract1/2
  Subtract2/1 -> If/1
  Constant4/1 -> Subtract2/1
  Square/1 -> Gain2/1
  Divide1/1 -> If/2
  Gain1/1 -> Divide1/2
  Constant5/1 -> Gain1/1
  If/1 -> If Action Subsystem4/Action
  Constant6/1 -> If Action Subsystem4/1(In1)
  If Action Subsystem4/1(Out1) -> Merge1/1
  If Action Subsystem4/2(Dec Override control) -> Merge/1
  Gain2/1 -> Divide1/1

== system Refined_Model_230322/Acceleration-Deceleration Driver/acc manoeuver1 ==
  In1 : Inport
  Action Port : ActionPort  ActionPortLabel=if(u1 > 0)
  Out1 : Outport
  wires:
  In1/1 -> Out1/1

== system Refined_Model_230322/Acceleration-Deceleration Driver/acc manoeuver2 ==
  In1 : Inport
  Action Port : ActionPort  ActionPortLabel=else
  Out1 : Outport
  wires:
  In1/1 -> Out1/1

== system Refined_Model_230322/Acceleration-Deceleration Driver/braking manoeuver1 ==
  In1 : Inport
  Action Port : ActionPort  ActionPortLabel=else
  Out1 : Outport
  wires:
  In1/1 -> Out1/1

== system Refined_Model_230322/Acceleration-Deceleration Driver/braking manoeuver2 ==
  In1 : Inport
  Action Port : ActionPort  ActionPortLabel=if(u1 < 0)
  Out1 : Outport
  wires:
  In1/1 -> Out1/1

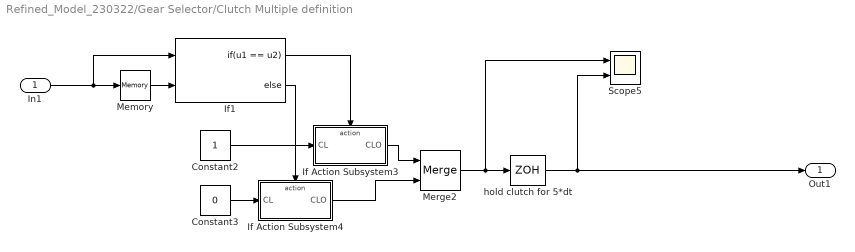
== system Refined_Model_230322/Gear Selector/Clutch Multiple definition ==
  In1 : Inport
  Constant2 : Constant
  Constant3 : Constant  Value=0
  If Action Subsystem3 : Subsystem  TreatAsAtomicUnit=on
  If Action Subsystem4 : Subsystem  TreatAsAtomicUnit=on
  If1 : If  NumInputs=2  IfExpression=u1 == u2
  Memory : Memory
  Merge2 : Merge
  Scope5 : Scope  NumInputPorts=2
  hold clutch for 5*dt : ZeroOrderHold  SampleTime=3*dt
  Out1 : Outport
  wires:
  If1/1 -> If Action Subsystem3/Action
  If Action Subsystem3/1(CLO) -> Merge2/1
  Memory/1 -> If1/2
  Constant2/1 -> If Action Subsystem3/1(CL)
  Constant3/1 -> If Action Subsystem4/1(CL)
  In1/1 -> Memory/1, If1/1
  If1/2 -> If Action Subsystem4/Action
  If Action Subsystem4/1(CLO) -> Merge2/2
  hold clutch for 5*dt/1 -> Scope5/2, Out1/1
  Merge2/1 -> Scope5/1, hold clutch for 5*dt/1

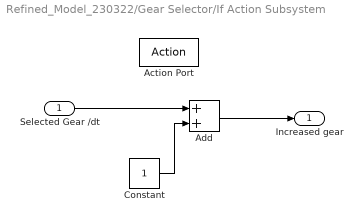
== system Refined_Model_230322/Gear Selector/If Action Subsystem ==
  Selected Gear /dt : Inport
  Action Port : ActionPort  ActionPortLabel=if(u1 >= u2 & u3 < u4)
  Add : Sum
  Constant : Constant
  Increased gear : Outport
  wires:
  Selected Gear /dt/1 -> Add/1
  Add/1 -> Increased gear/1
  Constant/1 -> Add/2

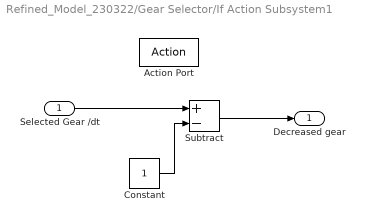
== system Refined_Model_230322/Gear Selector/If Action Subsystem1 ==
  Selected Gear /dt : Inport
  Action Port : ActionPort  ActionPortLabel=elseif(u3 >= u4 & u1 < u2)
  Constant : Constant
  Subtract : Sum  Inputs=+-
  Decreased gear : Outport
  wires:
  Constant/1 -> Subtract/2
  Subtract/1 -> Decreased gear/1
  Selected Gear /dt/1 -> Subtract/1

== system Refined_Model_230322/Gear Selector/If Action Subsystem2 ==
  Selected Gear Ratio /dt : Inport
  Action Port : ActionPort  ActionPortLabel=else
  Out1 : Outport
  wires:
  Selected Gear Ratio /dt/1 -> Out1/1

== system Refined_Model_230322/Vehicle Distance from Trip origin/If Action Subsystem ==
  In1 : Inport
  Action Port : ActionPort  ActionPortLabel=if(u1 > u2)
  Out1 : Outport
  wires:
  In1/1 -> Out1/1

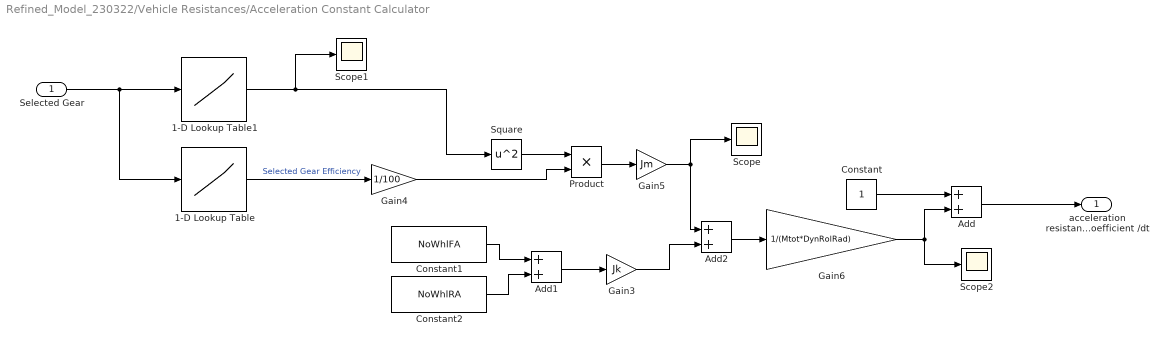
== system Refined_Model_230322/Vehicle Resistances/Acceleration Constant Calculator ==
  Selected Gear : Inport
  1-D Lookup Table : Lookup_n-D  NumberOfTableDimensions=1  BreakpointsForDimension1=GNo  Table=etaGRa  InternalRulePriority=Speed  RndMeth=Simplest  InputSameDT=on
  1-D Lookup Table1 : Lookup_n-D  NumberOfTableDimensions=1  BreakpointsForDimension1=GNo  Table=GRa  InternalRulePriority=Speed  RndMeth=Simplest  InputSameDT=on
  Add : Sum
  Add1 : Sum
  Add2 : Sum
  Constant : Constant
  Constant1 : Constant  Value=NoWhlFA
  Constant2 : Constant  Value=NoWhlRA
  Gain3 : Gain  Gain=Jk
  Gain4 : Gain  Gain=1/100
  Gain5 : Gain  Gain=Jm
  Gain6 : Gain  Gain=1/(Mtot*DynRolRad)
  Product : Product
  Scope : Scope
  Scope1 : Scope
  Scope2 : Scope
  Square : Math  Operator=square  SaturateOnIntegerOverflow=on
  acceleration resistance coefficient /dt : Outport
  wires:
  1-D Lookup Table/1 -> Gain4/1  "Selected Gear Efficiency"
  Add1/1 -> Gain3/1
  Product/1 -> Gain5/1
  Add/1 -> acceleration resistance coefficient /dt/1
  Gain6/1 -> Scope2/1, Add/2
  Square/1 -> Product/1
  Constant2/1 -> Add1/2
  Constant/1 -> Add/1
  Gain3/1 -> Add2/2
  Add2/1 -> Gain6/1
  Constant1/1 -> Add1/1
  Gain4/1 -> Product/2
  Gain5/1 -> Add2/1, Scope/1
  Selected Gear/1 -> 1-D Lookup Table/1, 1-D Lookup Table1/1
  1-D Lookup Table1/1 -> Scope1/1, Square/1

== system Refined_Model_230322/Acceleration-Deceleration Driver/Look Ahead Braking Model/If Action Subsystem ==
  In : Inport
  Action Port : ActionPort  ActionPortLabel=if(u1 > 0)
  1-D Lookup Table : Lookup_n-D  NumberOfTableDimensions=1  BreakpointsForDimension1=AccLim(:,1)  Table=AccLim(:,3)  InternalRulePriority=Speed  RndMeth=Simplest  InputSameDT=on
  Out1 : Outport
  wires:
  In/1 -> 1-D Lookup Table/1
  1-D Lookup Table/1 -> Out1/1  "deceleration in m/s^2"

== system Refined_Model_230322/Acceleration-Deceleration Driver/Look Ahead Braking Model/If Action Subsystem1 ==
  In1 : Inport
  Action Port : ActionPort  ActionPortLabel=else
  Out1 : Outport
  wires:
  In1/1 -> Out1/1

== system Refined_Model_230322/Acceleration-Deceleration Driver/Look Ahead Braking Model/If Action Subsystem2 ==
  In1 : Inport
  Action Port : ActionPort  ActionPortLabel=if(u1 <= u2 & u3 < u4)
  Out1 : Outport
  wires:
  In1/1 -> Out1/1

== system Refined_Model_230322/Acceleration-Deceleration Driver/Look Ahead Braking Model/If Action Subsystem3 ==
  In1 : Inport
  Action Port : ActionPort  ActionPortLabel=else
  Out1 : Outport
  wires:
  In1/1 -> Out1/1

== system Refined_Model_230322/Acceleration-Deceleration Driver/Look Ahead Braking Model/If Action Subsystem4 ==
  In1 : Inport
  Action Port : ActionPort  ActionPortLabel=if(u1 == u2)
  Constant : Constant
  Out1 : Outport
  Dec Override control : Outport  Port=2
  wires:
  In1/1 -> Out1/1
  Constant/1 -> Dec Override control/1

== system Refined_Model_230322/Gear Selector/Clutch Multiple definition/If Action Subsystem3 ==
  CL : Inport
  Action Port : ActionPort  ActionPortLabel=if(u1 == u2)
  CLO : Outport
  wires:
  CL/1 -> CLO/1

== system Refined_Model_230322/Gear Selector/Clutch Multiple definition/If Action Subsystem4 ==
  CL : Inport
  Action Port : ActionPort  ActionPortLabel=else
  CLO : Outport
  wires:
  CL/1 -> CLO/1
